simulink model "foc"  (R2021b)
settings: Solver=FixedStepAuto  StartTime=0.0  StopTime=20  FixedStep=Ts  MaxStep=1e-4  RelTol=1e-3  EnableMultiTasking=on
model workspace (MAT data in the model file):
  flux = 0.154
values from neighbouring files (symbols this model uses):
  currt_width = 200.0    [motor_parameters.sldd]
  Flux = 0.00103001    [motor_parameters.sldd]
  Ibus = 5.0    [motor_parameters.sldd]
  Ld = 2.235E-5    [motor_parameters.sldd]
  Lq = 2.567E-5    [motor_parameters.sldd]
  Ls = 2.235E-5    [motor_parameters.sldd]
  OPL_time = 3.0    [motor_parameters.sldd]
  Pn = 7.0    [motor_parameters.sldd]
  R = 0.083    [motor_parameters.sldd]
  Rs = 0.112    [motor_parameters.sldd]
  smo_l = 0.1    [motor_parameters.sldd]
  smo_m = 0.001    [motor_parameters.sldd]
  Ts = 0.0001    [motor_parameters.sldd]
  Ubus = 12.0    [motor_parameters.sldd]
undefined symbols (not defined in the file or in its folder): DiscIntNeverNeededParam, sigbuilder_block, spd_ki, spd_kp
libraries: slpidlib x6, simulink x3, mcbcontrolslib x3, mcbplantlib x1, autolibpmsmexterior x1
(part 2 of 2)

== system foc/FOC_Model/currloop/HFI_Observer/waichafa ==
  i_alpha_n : Inport
  i_beta_n : Inport  Port=2
  "   " : Product
  "    " : Product
  Discrete PID Controller : slpidlib/PID Controller  Controller=PI  Form=Parallel  TimeDomain=Discrete-time  UseExternalTs=off  SampleTime=-1  IntegratorMethod=Forward Euler  FilterMethod=Forward Euler  ControllerParametersSource=internal  P=100  I=15000  D=0  UseFilter=on  N=100  TunerSelectOption=Transfer Function Based (PID Tuner App)  InitialConditionSource=internal  InitialConditionForIntegrator=0  InitialConditionForFilter=0  DifferentiatorICPrevScaledInput=0  ExternalReset=none  TrackingMode=off  Kt=1  LimitOutput=off  SatLimitsSource=internal  UpperSaturationLimit=inf  LowerSaturationLimit=-inf  LinearizeAsGain=off  AntiWindupMode=none  Kb=1  POutMin=[]  POutMax=[]  IOutMin=[]  IOutMax=[]  DOutMin=[]  DOutMax=[]  NOutMin=[]  NOutMax=[]  SumOutMin=[]  SumOutMax=[]  SaturationOutMin=[]  SaturationOutMax=[]  PParamMin=[]  PParamMax=[]  IParamMin=[]  IParamMax=[]  DParamMin=[]  DParamMax=[]  NParamMin=[]  NParamMax=[]  KbParamMin=[]  KbParamMax=[]  KtParamMin=[]  KtParamMax=[]  KbOutMin=[]  KbOutMax=[]  KtOutMin=[]  KtOutMax=[]  IntegratorOutMin=[]  IntegratorOutMax=[]  FilterOutMin=[]  FilterOutMax=[]  SumI1OutMin=[]  SumI1OutMax=[]  SumI2OutMin=[]  SumI2OutMax=[]  SumI3OutMin=[]  SumI3OutMax=[]  SumI4OutMin=[]  SumI4OutMax=[]  SumDOutMin=[]  SumDOutMax=[]  DifferentiatorOutMin=[]  DifferentiatorOutMax=[]  FilterDiffOutCoefMin=[]  FilterDiffOutCoefMax=[]  ReciprocalOutMin=[]  ReciprocalOutMax=[]  SumDenOutMin=[]  SumDenOutMax=[]  SumNumOutMin=[]  SumNumOutMax=[]  DivideOutMin=[]  DivideOutMax=[]  UdiffTsProdOutMin=[]  UdiffTsProdOutMax=[]  NTsProdOutMin=[]  NTsProdOutMax=[]  UintegralTsProdOutMin=[]  UintegralTsProdOutMax=[]  UngainTsProdOutMin=[]  UngainTsProdOutMax=[]  IntegratorContinuousStateAttributes=''  IntegratorStateMustResolveToSignalObject=off  IntegratorRTWStateStorageClass=Auto  FilterContinuousStateAttributes=''  FilterStateMustResolveToSignalObject=off  FilterRTWStateStorageClass=Auto  ParallelPVariant=InternalParameters  IdealPVariant=Disabled  IVariant=InternalParameters  DVariant=Disabled  IntegratorVariant=Discrete  SatVariant=Disabled  AWVariant=Passthrough  PCopyVariant=Disabled  TRVariant=Disabled  FdbkBlocksVariant=Forward  IdealPFdbkVariant=Disabled  SatFdbkVariant=Disabled  DerivativeFilterVariant=Disabled  NVariant=Disabled  NCopyVariant=Disabled_SignalSpec  FilterICVariant=Disabled  IntegratorICVariant=InternalICs  ExternalResetVariant=Disabled  TRSumVariant=Passthrough  SumFdbkVariant=Disabled  SumVariant=Sum_PI  TsampFilterVariant=InternalTs  TsampNgainVariant=Passthrough  TsampIntegralVariant=Passthrough  ExternalSaturationOutDataTypeStr=Inherit: Same as second input
  Discrete-Time Integrator : DiscreteIntegrator  SampleTime=-1  ICPrevOutput=DiscIntNeverNeededParam  ICPrevScaledInput=DiscIntNeverNeededParam
  Fcn : Fcn  Expr=sin(u(1))
  Fcn1 : Fcn  Expr=cos(u(1))
  Fcn2 : Fcn  Expr=u(1)/sqrt(u(1)*u(1)+u(2)*u(2))
  Fcn3 : Fcn  Expr=u(2)/sqrt(u(1)*u(1)+u(2)*u(2))
  Mux : Mux  Inputs=2
  Scope : Scope  NumInputPorts=2
  Scope1 : Scope
  Sum9 : Sum  Inputs=-+
  theta : Outport  VectorParamsAs1DForOutWhenUnconnected=off
  we : Outport  Port=2  VectorParamsAs1DForOutWhenUnconnected=off
  wires:
  "   "/1 -> Sum9/2
  Fcn1/1 -> "   "/1
  "    "/1 -> Sum9/1
  Fcn/1 -> "    "/2
  i_alpha_n/1 -> Mux/1
  Mux/1 -> Fcn3/1, Fcn2/1
  Fcn2/1 -> Scope/1, "    "/1
  Discrete-Time Integrator/1 -> theta/1, Fcn/1, Fcn1/1
  Fcn3/1 -> "   "/2, Scope/2
  Sum9/1 -> Scope1/1, Discrete PID Controller/1
  Discrete PID Controller/1 -> we/1, Discrete-Time Integrator/1
  i_beta_n/1 -> Mux/2

== system foc/FOC_Model/currloop/If Action Subsystem2/If Action Subsystem ==
  Action Port : ActionPort  ActionPortLabel=if(u1 >= 0)
  Constant : Constant  Value=0  OutDataTypeStr=single
  Out1 : Outport
  wires:
  Constant/1 -> Out1/1

== system foc/FOC_Model/currloop/If Action Subsystem2/If Action Subsystem1 ==
  Action Port : ActionPort  ActionPortLabel=else
  Constant : Constant  Value=pi  OutDataTypeStr=single
  Out1 : Outport
  wires:
  Constant/1 -> Out1/1

== system foc/FOC_Model/currloop/SMO/PLL ==
  e_alpha_est : Inport
  e_beta_est : Inport  Port=2
  Constant : Constant  Value=2*pi  SampleTime=-1
  Cos : Trigonometry  Operator=cos
  Discrete-Time Integrator : DiscreteIntegrator  SampleTime=-1  ICPrevOutput=DiscIntNeverNeededParam  ICPrevScaledInput=DiscIntNeverNeededParam
  IIR Filter : mcbcontrolslib/IIR Filter  VariantControl=Low Pass Filter  VariantSelect=Low-pass  Filter_constant=0.0004  advancedSettings=on  Ts=1e-6  cutOff_freq=63.6875
      settings: SourceProductBaseCode=MT
  IIR Filter1 : mcbcontrolslib/IIR Filter  VariantControl=Low Pass Filter  VariantSelect=Low-pass  Filter_constant=0.0004  advancedSettings=on  Ts=1e-5  cutOff_freq=6.3687
      settings: SourceProductBaseCode=MT
  Mod : Math  Operator=mod  SaturateOnIntegerOverflow=on
  PLL : Subsystem
      mask Display: disp('PI')
  Product : Product
  Product1 : Product
  Scope : Scope
  Sin : Trigonometry
  Sum : Sum  Inputs=--
  theta_est : Outport
  we_est : Outport  Port=2
  wires:
  e_alpha_est/1 -> Product/2
  Cos/1 -> Product/1
  Product/1 -> Sum/1
  e_beta_est/1 -> Product1/1
  Product1/1 -> Sum/2
  Sin/1 -> Product1/2
  Discrete-Time Integrator/1 -> Mod/1, Cos/1, Sin/1
  Sum/1 -> PLL/1(e)
  PLL/1(output) -> IIR Filter1/1, Discrete-Time Integrator/1
  IIR Filter1/1 -> Scope/1, we_est/1
  Mod/1 -> theta_est/1
  Constant/1 -> Mod/2

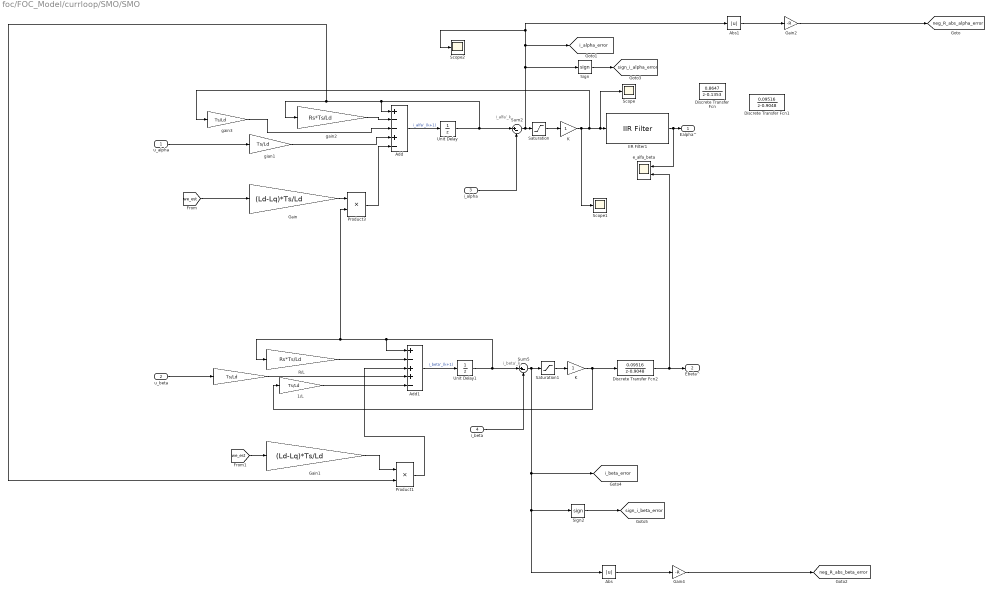
== system foc/FOC_Model/currloop/SMO/SMO ==
  note: i_alfa'_k
  note: i_beta'_k
  u_alpha : Inport  OutDataTypeStr=single
  u_beta : Inport  Port=2  OutDataTypeStr=single
  i_alpha : Inport  Port=3  OutDataTypeStr=single
  i_beta : Inport  Port=4  OutDataTypeStr=single
  " " : Gain  Gain=Ts/Ld
  " 1/L " : Gain  Gain=Ts/Ld
  Abs : Abs
  Abs1 : Abs
  Add : Sum  Inputs=+--+-  OutDataTypeStr=single
  Add1 : Sum  Inputs=+-++-
  Discrete Transfer Fcn : DiscreteTransferFcn  Numerator=[0.8647]  Denominator=[1 -0.1353]
  Discrete Transfer Fcn1 : DiscreteTransferFcn  Numerator=[0.09516]  Denominator=[1 -0.9048]
  Discrete Transfer Fcn2 : DiscreteTransferFcn  Numerator=[0.09516]  Denominator=[1 -0.9048]
  Gain : Gain  Gain=(Ld-Lq)*Ts/Ld
  Gain1 : Gain  Gain=(Ld-Lq)*Ts/Ld
  Gain2 : Gain  Gain=-R
  Gain4 : Gain  Gain=-R
  IIR Filter1 : mcbcontrolslib/IIR Filter  VariantControl=Low Pass Filter  VariantSelect=Low-pass  Filter_constant=0.1  advancedSettings=on  Ts=1e-4  cutOff_freq=176.8388
      settings: SourceProductBaseCode=MT
  K : Gain
  "K " : Gain
  Product1 : Product  RndMeth=Zero
  Product3 : Product  RndMeth=Zero
  "R/L " : Gain  Gain=Rs*Ts/Ld
  Saturation : Saturate  UpperLimit=2  LowerLimit=-2
  Saturation1 : Saturate  UpperLimit=2  LowerLimit=-2
  Scope : Scope
  Scope1 : Scope
  Scope2 : Scope
  Sign : Signum  ZeroCross=off
  Sign2 : Signum  ZeroCross=off
  Sum2 : Sum  Inputs=|+-
  Sum5 : Sum  Inputs=|+-
  Unit Delay : UnitDelay  SampleTime=-1  HasFrameUpgradeWarning=on
  Unit Delay1 : UnitDelay  SampleTime=-1  HasFrameUpgradeWarning=on
  e_alfa_beta : Scope  NumInputPorts=2
  gain2 : Gain  Gain=Rs*Ts/Ld  OutDataTypeStr=single
  gain3 : Gain  Gain=Ts/Ld
  gian1 : Gain  Gain=Ts/Ld
  Ealpha^ : Outport
  Ebeta^ : Outport  Port=2
  tag scope: i_alpha_error=global, i_beta_error=global, neg_R_abs_alpha_error=global, neg_R_abs_beta_error=global, sign_i_alpha_error=global, sign_i_beta_error=global
  wires:
  Saturation/1 -> K/1
  K/1 -> Scope1/1, IIR Filter1/1, Scope/1, gain3/1
  Unit Delay1/1 -> Add1/1, Product3/2, "R/L "/1, Sum5/1
  Saturation1/1 -> "K "/1
  " "/1 -> Add1/4
  "R/L "/1 -> Add1/2
  [we_est] -> Gain/1
  Gain/1 -> Product3/1
  Gain1/1 -> Product1/1
  [we_est] -> Gain1/1
  Product1/1 -> Add1/3
  Unit Delay/1 -> Product1/2, gain2/1, Add/1, Sum2/1
  Add/1 -> Unit Delay/1  "i_alfa'_(k+1)"
  gain2/1 -> Add/2
  gian1/1 -> Add/4
  Product3/1 -> Add/5
  gain3/1 -> Add/3
  Add1/1 -> Unit Delay1/1  "i_beta'_(k+1)"
  " 1/L "/1 -> Add1/5
  Sum2/1 -> Sign/1, [i_alpha_error], Scope2/1, Abs1/1, Saturation/1
  Gain2/1 -> [neg_R_abs_alpha_error]
  Abs1/1 -> Gain2/1
  Abs/1 -> Gain4/1
  Gain4/1 -> [neg_R_abs_beta_error]
  Sum5/1 -> Sign2/1, Abs/1, [i_beta_error], Saturation1/1
  Sign/1 -> [sign_i_alpha_error]
  Sign2/1 -> [sign_i_beta_error]
  u_alpha/1 -> gian1/1
  u_beta/1 -> " "/1
  i_alpha/1 -> Sum2/2
  i_beta/1 -> Sum5/2
  "K "/1 -> Discrete Transfer Fcn2/1, " 1/L "/1
  Discrete Transfer Fcn2/1 -> e_alfa_beta/2, Ebeta^/1
  IIR Filter1/1 -> e_alfa_beta/1, Ealpha^/1

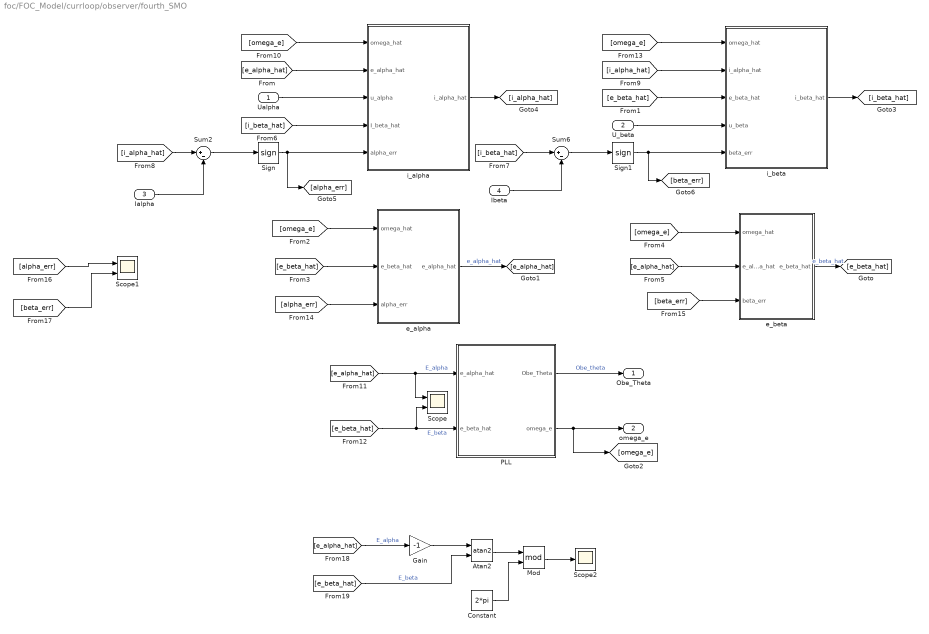
== system foc/FOC_Model/currloop/observer/fourth_SMO ==
  Ualpha : Inport
  U_beta : Inport  Port=2
  Ialpha : Inport  Port=3
  Ibeta : Inport  Port=4
  Atan2 : Trigonometry  Operator=atan2
  Constant : Constant  Value=2*pi  OutDataTypeStr=single
  Gain : Gain  Gain=-1  OutDataTypeStr=single
  Mod : Math  Operator=mod  SaturateOnIntegerOverflow=on
  PLL : Subsystem
  Scope : Scope  NumInputPorts=2
  Scope1 : Scope  NumInputPorts=2
  Scope2 : Scope
  Sign : Signum
  Sign1 : Signum
  Sum2 : Sum  Inputs=|+-
  Sum6 : Sum  Inputs=|+-
  e_alpha : Subsystem
  e_beta : Subsystem
  i_alpha : Subsystem
  i_beta : Subsystem
  Obe_Theta : Outport
  omega_e : Outport  Port=2
  wires:
  Sum6/1 -> Sign1/1
  Sum2/1 -> Sign/1
  Sign/1 -> i_alpha/5(alpha_err), [alpha_err]
  Ialpha/1 -> Sum2/2
  Sign1/1 -> [beta_err], i_beta/5(beta_err)
  Ibeta/1 -> Sum6/2
  i_alpha/1(i_alpha_hat) -> [i_alpha_hat]
  [e_alpha_hat] -> i_alpha/2(e_alpha_hat)
  Ualpha/1 -> i_alpha/3(u_alpha)
  [e_beta_hat] -> i_beta/3(e_beta_hat)
  U_beta/1 -> i_beta/4(u_beta)
  i_beta/1(i_beta_hat) -> [i_beta_hat]
  [i_beta_hat] -> i_alpha/4(I_beta_hat)
  [i_beta_hat] -> Sum6/1
  [i_alpha_hat] -> Sum2/1
  [i_alpha_hat] -> i_beta/2(i_alpha_hat)
  [omega_e] -> e_alpha/1(omega_hat)
  [e_beta_hat] -> e_alpha/2(e_beta_hat)
  [omega_e] -> e_beta/1(omega_hat)
  [e_alpha_hat] -> e_beta/2(e_alpha_hat)
  [omega_e] -> i_alpha/1(omega_hat)
  e_beta/1(e_beta_hat) -> [e_beta_hat]  "e_beta_hat"
  e_alpha/1(e_alpha_hat) -> [e_alpha_hat]  "e_alpha_hat"
  [e_alpha_hat] -> Scope/1, PLL/1(e_alpha_hat)  "E_alpha"
  [e_beta_hat] -> Scope/2, PLL/2(e_beta_hat)  "E_beta"
  PLL/2(omega_e) -> [omega_e], omega_e/1
  [omega_e] -> i_beta/1(omega_hat)
  PLL/1(Obe_Theta) -> Obe_Theta/1  "Obe_theta"
  [alpha_err] -> e_alpha/3(alpha_err)
  [beta_err] -> e_beta/3(beta_err)
  [alpha_err] -> Scope1/1
  [beta_err] -> Scope1/2
  [e_alpha_hat] -> Gain/1  "E_alpha"
  Gain/1 -> Atan2/1
  [e_beta_hat] -> Atan2/2  "E_beta"
  Atan2/1 -> Mod/1
  Constant/1 -> Mod/2
  Mod/1 -> Scope2/1

== system foc/FOC_Model/currloop/svpwm/Anti_Park_Trans ==
  note: Valpha = ud*cos(theta) - uq*sin(theta);
      | Vbeta = ud*sin(theta) + uq*cos(theta);
  ud : Inport  OutDataTypeStr=single
  uq : Inport  Port=2  OutDataTypeStr=single
  theta : Inport  Port=3
  Add : Sum  Inputs=+-
  Add1 : Sum
  Cos : Trigonometry  Operator=cos
  Product{,1..3} (4 alike) : Product
  Scope : Scope  NumInputPorts=2
  Sin : Trigonometry
  ualpha : Outport  OutDataTypeStr=single
  ubeta : Outport  Port=2  OutDataTypeStr=single
  wires:
  Add/1 -> ualpha/1
  ud/1 -> Product2/1, Product/1
  Cos/1 -> Product/2, Scope/2, Product3/2
  Product/1 -> Add/1
  uq/1 -> Product3/1, Product1/1
  theta/1 -> Sin/1, Cos/1
  Product1/1 -> Add/2
  Product2/1 -> Add1/1
  Product3/1 -> Add1/2
  Add1/1 -> ubeta/1
  Sin/1 -> Scope/1, Product2/2, Product1/2

== system foc/FOC_Model/currloop/SMO/PLL/PLL ==
  e : Inport
  Add : Sum
  Discrete-Time Integrator : DiscreteIntegrator  SampleTime=-1  ICPrevOutput=DiscIntNeverNeededParam  ICPrevScaledInput=DiscIntNeverNeededParam
  Ki : Gain  Gain=36000
  Kp : Gain  Gain=540
  Saturation : Saturate  UpperLimit=2000  LowerLimit=-2000
  output : Outport
  wires:
  Ki/1 -> Discrete-Time Integrator/1
  e/1 -> Kp/1, Ki/1
  Saturation/1 -> output/1
  Discrete-Time Integrator/1 -> Add/2
  Kp/1 -> Add/1
  Add/1 -> Saturation/1

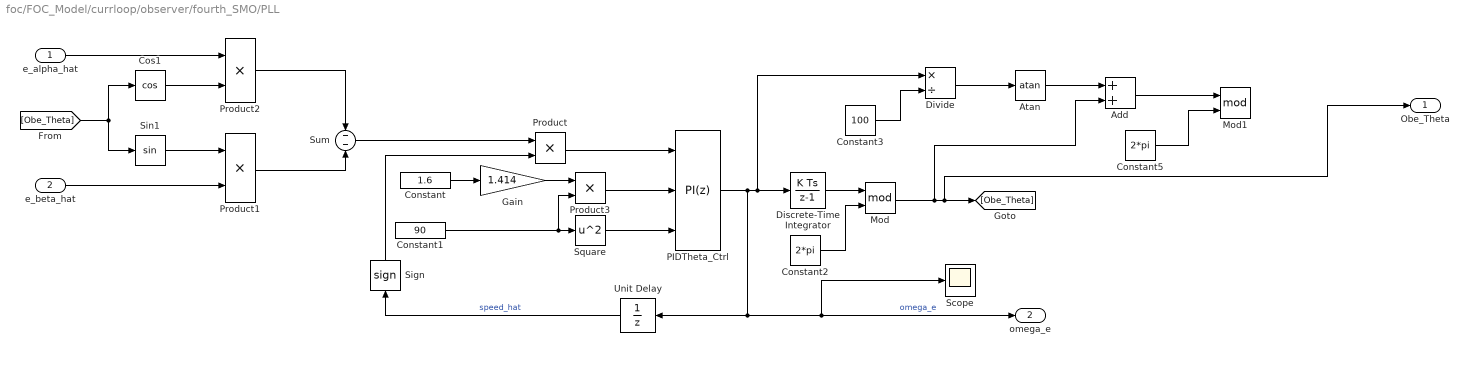
== system foc/FOC_Model/currloop/observer/fourth_SMO/PLL ==
  e_alpha_hat : Inport
  e_beta_hat : Inport  Port=2
  Add : Sum
  Atan : Trigonometry  Operator=atan
  Constant : Constant  Value=1.6  OutDataTypeStr=single  SampleTime=-1
  Constant1 : Constant  Value=90  OutDataTypeStr=single  SampleTime=-1
  Constant2 : Constant  Value=2*pi  OutDataTypeStr=single  SampleTime=Ts
  Constant3 : Constant  Value=100
  Constant5 : Constant  Value=2*pi  OutDataTypeStr=single  SampleTime=Ts
  Cos1 : Trigonometry  Operator=cos
  Discrete-Time Integrator : DiscreteIntegrator  SampleTime=Ts  ICPrevOutput=DiscIntNeverNeededParam  ICPrevScaledInput=DiscIntNeverNeededParam
  Divide : Product  Inputs=*/  OutDataTypeStr=single
  Gain : Gain  Gain=1.414
  Mod : Math  Operator=mod  SignedPower=on  SaturateOnIntegerOverflow=on
  Mod1 : Math  Operator=mod  SaturateOnIntegerOverflow=on
  PIDTheta_Ctrl : slpidlib/PID Controller  Controller=PI  Form=Parallel  TimeDomain=Discrete-time  UseExternalTs=off  SampleTime=-1  IntegratorMethod=Forward Euler  FilterMethod=Forward Euler  ControllerParametersSource=external  P=2*0.707*100  I=100*100  D=0  UseFilter=on  N=100  TunerSelectOption=Transfer Function Based (PID Tuner App)  ZeroCross=off  InitialConditionSource=internal  InitialConditionForIntegrator=50  InitialConditionForFilter=0  DifferentiatorICPrevScaledInput=0  ExternalReset=none  TrackingMode=off  Kt=1  LimitOutput=on  SatLimitsSource=internal  UpperSaturationLimit=3000  LowerSaturationLimit=-3000  LinearizeAsGain=off  AntiWindupMode=clamping  Kb=50  POutMin=[]  POutMax=[]  IOutMin=[]  IOutMax=[]  DOutMin=[]  DOutMax=[]  NOutMin=[]  NOutMax=[]  SumOutMin=[]  SumOutMax=[]  SaturationOutDataTypeStr=Inherit: Inherit via back propagation  SaturationOutMin=[]  SaturationOutMax=[]  PParamMin=[]  PParamMax=[]  IParamMin=[]  IParamMax=[]  DParamMin=[]  DParamMax=[]  NParamMin=[]  NParamMax=[]  KbParamMin=[]  KbParamMax=[]  KtParamMin=[]  KtParamMax=[]  KbOutMin=[]  KbOutMax=[]  KtOutMin=[]  KtOutMax=[]  IntegratorOutMin=[]  IntegratorOutMax=[]  FilterOutMin=[]  FilterOutMax=[]  SumI1OutMin=[]  SumI1OutMax=[]  SumI2OutMin=[]  SumI2OutMax=[]  SumI3OutMin=[]  SumI3OutMax=[]  SumI4OutMin=[]  SumI4OutMax=[]  SumDOutMin=[]  SumDOutMax=[]  DifferentiatorOutMin=[]  DifferentiatorOutMax=[]  FilterDiffOutCoefMin=[]  FilterDiffOutCoefMax=[]  ReciprocalOutMin=[]  ReciprocalOutMax=[]  SumDenOutMin=[]  SumDenOutMax=[]  SumNumOutMin=[]  SumNumOutMax=[]  DivideOutMin=[]  DivideOutMax=[]  UdiffTsProdOutMin=[]  UdiffTsProdOutMax=[]  NTsProdOutMin=[]  NTsProdOutMax=[]  UintegralTsProdOutMin=[]  UintegralTsProdOutMax=[]  UngainTsProdOutMin=[]  UngainTsProdOutMax=[]  IntegratorContinuousStateAttributes=''  IntegratorStateMustResolveToSignalObject=off  IntegratorRTWStateStorageClass=Auto  FilterContinuousStateAttributes=''  FilterStateMustResolveToSignalObject=off  FilterRTWStateStorageClass=Auto  ParallelPVariant=ExternalParameters  IdealPVariant=Disabled  IVariant=ExternalParameters  DVariant=Disabled  IntegratorVariant=Discrete  SatVariant=Enabled  AWVariant=DiscClampingParallel  PCopyVariant=Disabled  TRVariant=Disabled  FdbkBlocksVariant=Forward  IdealPFdbkVariant=Disabled  SatFdbkVariant=Disabled  DerivativeFilterVariant=Disabled  NVariant=Disabled  NCopyVariant=Disabled_SignalSpec  FilterICVariant=Disabled  IntegratorICVariant=InternalICs  ExternalResetVariant=Disabled  TRSumVariant=Passthrough  SumFdbkVariant=Disabled  SumVariant=Sum_PI  TsampFilterVariant=InternalTs  TsampNgainVariant=Passthrough  TsampIntegralVariant=Passthrough  ExternalSaturationOutDataTypeStr=Inherit: Same as second input
  Product{,1..3} (4 alike) : Product
  Scope : Scope
  Sign : Signum
  Sin1 : Trigonometry
  Square : Math  Operator=square  SignedPower=on  SaturateOnIntegerOverflow=on
  Sum : Sum  Inputs=-|-
  Unit Delay : UnitDelay  SampleTime=-1  HasFrameUpgradeWarning=on
  Obe_Theta : Outport
  omega_e : Outport  Port=2
  wires:
  Product/1 -> PIDTheta_Ctrl/1
  Sum/1 -> Product/1
  Product1/1 -> Sum/2
  Product2/1 -> Sum/1
  Unit Delay/1 -> Sign/1  "speed_hat"
  Sign/1 -> Product/2
  PIDTheta_Ctrl/1 -> Divide/1, Discrete-Time Integrator/1, Scope/1, omega_e/1, Unit Delay/1  "omega_e"
  Constant/1 -> Gain/1
  Constant1/1 -> Product3/2, Square/1
  Square/1 -> PIDTheta_Ctrl/3
  Gain/1 -> Product3/1
  Product3/1 -> PIDTheta_Ctrl/2
  Mod/1 -> Obe_Theta/1, [Obe_Theta], Add/2
  Discrete-Time Integrator/1 -> Mod/1
  Constant2/1 -> Mod/2
  e_alpha_hat/1 -> Product2/1
  Cos1/1 -> Product2/2
  Sin1/1 -> Product1/1
  e_beta_hat/1 -> Product1/2
  Constant3/1 -> Divide/2
  Divide/1 -> Atan/1
  Atan/1 -> Add/1
  Add/1 -> Mod1/1
  Constant5/1 -> Mod1/2
  [Obe_Theta] -> Cos1/1, Sin1/1

== system foc/FOC_Model/currloop/observer/fourth_SMO/e_alpha ==
  omega_hat : Inport
  e_beta_hat : Inport  Port=2
  alpha_err : Inport  Port=3
  Add2 : Sum  Inputs=-+
  Constant : Constant  Value=Ld  OutDataTypeStr=single
  Discrete-Time Integrator : DiscreteIntegrator  SampleTime=Ts  ICPrevOutput=DiscIntNeverNeededParam  ICPrevScaledInput=DiscIntNeverNeededParam
  Divide : Product  Inputs=*/
  Gain3 : Gain  Gain=smo_m
  Product2 : Product
  Unit Delay2 : UnitDelay  SampleTime=-1  HasFrameUpgradeWarning=on
  e_alpha_hat : Outport
  wires:
  Unit Delay2/1 -> e_alpha_hat/1
  omega_hat/1 -> Product2/1
  Product2/1 -> Add2/1
  Discrete-Time Integrator/1 -> Unit Delay2/1
  e_beta_hat/1 -> Product2/2
  Divide/1 -> Add2/2
  alpha_err/1 -> Gain3/1
  Constant/1 -> Divide/2
  Gain3/1 -> Divide/1
  Add2/1 -> Discrete-Time Integrator/1

== system foc/FOC_Model/currloop/observer/fourth_SMO/e_beta ==
  omega_hat : Inport
  e_alpha_hat : Inport  Port=2
  beta_err : Inport  Port=3
  Add3 : Sum
  Constant : Constant  Value=Ld  OutDataTypeStr=single
  Discrete-Time Integrator : DiscreteIntegrator  SampleTime=Ts  ICPrevOutput=DiscIntNeverNeededParam  ICPrevScaledInput=DiscIntNeverNeededParam
  Divide : Product  Inputs=*/
  Gain1 : Gain  Gain=smo_m
  Product3 : Product
  Unit Delay3 : UnitDelay  SampleTime=-1  HasFrameUpgradeWarning=on
  e_beta_hat : Outport
  wires:
  Discrete-Time Integrator/1 -> Unit Delay3/1
  Product3/1 -> Add3/1
  Unit Delay3/1 -> e_beta_hat/1
  omega_hat/1 -> Product3/1
  e_alpha_hat/1 -> Product3/2
  Constant/1 -> Divide/2
  beta_err/1 -> Gain1/1
  Divide/1 -> Add3/2
  Gain1/1 -> Divide/1
  Add3/1 -> Discrete-Time Integrator/1

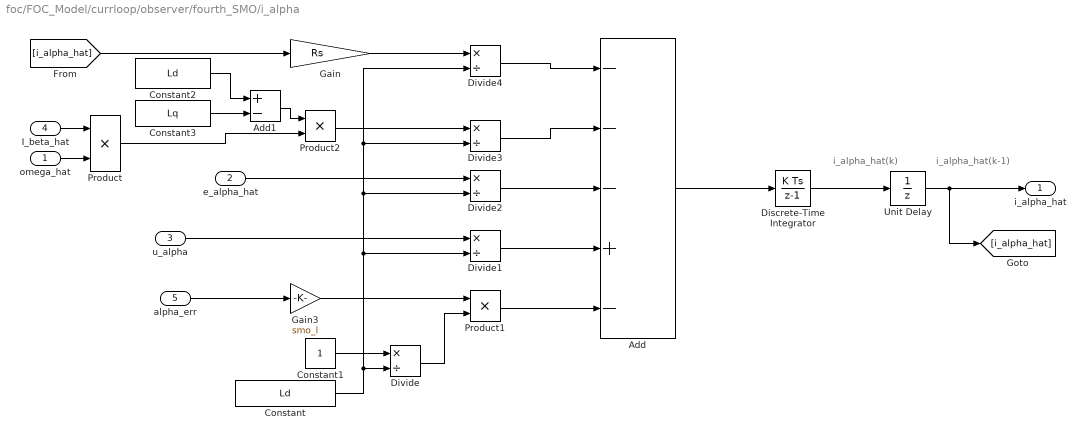
== system foc/FOC_Model/currloop/observer/fourth_SMO/i_alpha ==
  note: i_alpha_hat(k)
  note: i_alpha_hat(k-1)
  omega_hat : Inport
  e_alpha_hat : Inport  Port=2
  u_alpha : Inport  Port=3
  I_beta_hat : Inport  Port=4
  alpha_err : Inport  Port=5
  Add : Sum  Inputs=---+-
  Add1 : Sum  Inputs=+-
  Constant : Constant  Value=Ld  OutDataTypeStr=single
  Constant1 : Constant  OutDataTypeStr=single
  Constant2 : Constant  Value=Ld  OutDataTypeStr=single
  Constant3 : Constant  Value=Lq  OutDataTypeStr=single
  Discrete-Time Integrator : DiscreteIntegrator  SampleTime=Ts  ICPrevOutput=DiscIntNeverNeededParam  ICPrevScaledInput=DiscIntNeverNeededParam
  Divide{,1..4} (5 alike) : Product  Inputs=*/
  Gain : Gain  Gain=Rs
  Gain3 : Gain  Gain=smo_l
  Product : Product
  Product1 : Product
  Product2 : Product
  Unit Delay : UnitDelay  SampleTime=-1  HasFrameUpgradeWarning=on
  i_alpha_hat : Outport
  wires:
  Divide3/1 -> Add/2
  Product1/1 -> Add/5
  Add/1 -> Discrete-Time Integrator/1
  I_beta_hat/1 -> Product/1
  Unit Delay/1 -> [i_alpha_hat], i_alpha_hat/1
  u_alpha/1 -> Divide1/1
  Divide1/1 -> Add/4
  Discrete-Time Integrator/1 -> Unit Delay/1
  omega_hat/1 -> Product/2
  Divide2/1 -> Add/3
  e_alpha_hat/1 -> Divide2/1
  alpha_err/1 -> Gain3/1
  [i_alpha_hat] -> Gain/1
  Gain3/1 -> Product1/1
  Constant/1 -> Divide2/2, Divide3/2, Divide4/2, Divide1/2, Divide/2
  Divide/1 -> Product1/2
  Constant1/1 -> Divide/1
  Constant2/1 -> Add1/1
  Constant3/1 -> Add1/2
  Product/1 -> Product2/2
  Add1/1 -> Product2/1
  Product2/1 -> Divide3/1
  Divide4/1 -> Add/1
  Gain/1 -> Divide4/1

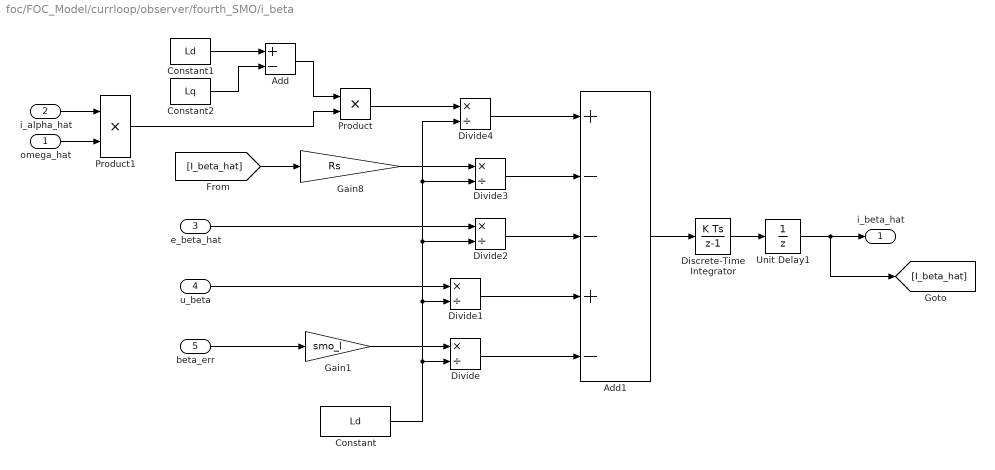
== system foc/FOC_Model/currloop/observer/fourth_SMO/i_beta ==
  omega_hat : Inport
  i_alpha_hat : Inport  Port=2
  e_beta_hat : Inport  Port=3
  u_beta : Inport  Port=4
  beta_err : Inport  Port=5
  Add : Sum  Inputs=+-
  Add1 : Sum  Inputs=+--+-
  Constant : Constant  Value=Ld  OutDataTypeStr=single
  Constant1 : Constant  Value=Ld  OutDataTypeStr=single
  Constant2 : Constant  Value=Lq  OutDataTypeStr=single
  Discrete-Time Integrator : DiscreteIntegrator  SampleTime=Ts  ICPrevOutput=DiscIntNeverNeededParam  ICPrevScaledInput=DiscIntNeverNeededParam
  Divide{,1..4} (5 alike) : Product  Inputs=*/
  Gain1 : Gain  Gain=smo_l
  Gain8 : Gain  Gain=Rs
  Product : Product
  Product1 : Product
  Unit Delay1 : UnitDelay  SampleTime=-1  HasFrameUpgradeWarning=on
  i_beta_hat : Outport
  wires:
  u_beta/1 -> Divide1/1
  Add1/1 -> Discrete-Time Integrator/1
  i_alpha_hat/1 -> Product1/1
  Discrete-Time Integrator/1 -> Unit Delay1/1
  e_beta_hat/1 -> Divide2/1
  Unit Delay1/1 -> i_beta_hat/1, [I_beta_hat]
  omega_hat/1 -> Product1/2
  [I_beta_hat] -> Gain8/1
  Gain1/1 -> Divide/1
  beta_err/1 -> Gain1/1
  Divide/1 -> Add1/5
  Constant/1 -> Divide4/2, Divide3/2, Divide2/2, Divide1/2, Divide/2
  Divide1/1 -> Add1/4
  Divide2/1 -> Add1/3
  Divide3/1 -> Add1/2
  Gain8/1 -> Divide3/1
  Constant1/1 -> Add/1
  Constant2/1 -> Add/2
  Divide4/1 -> Add1/1
  Product/1 -> Divide4/1
  Product1/1 -> Product/2
  Add/1 -> Product/1

== matlab function foc/FOC_Model/currloop/svpwm/foc ==
  data: Valpha input; Tcmp1 output; Vbeta input; Udc input; Tpwm input; Tcmp2 output; Tcmp3 output; sector output
function [Tcmp1,Tcmp2,Tcmp3,sector] = fcn(Valpha,Vbeta,Udc,Tpwm)
%#codegen

sector = single(0);
Tcmp1 = single(0);
Tcmp2 = single(0);
Tcmp3 = single(0);

%========Parameters statement================

    Vref1 = Vbeta;							                   
    Vref2 = (sqrt(3)*Valpha - Vbeta)/2; 				    
    Vref3 = (-sqrt(3)*Valpha - Vbeta)/2;					
   
 %========Sector calculation=================

  if (Vref1>0)
	   sector = single(1);
  end
  if (Vref2>0)
	   sector = sector+single(2);
  end
  if (Vref3>0)
       sector = sector+single(4);
  end

%======== X Y Z calculation===================

X = sqrt(3)*Vbeta*Tpwm/Udc;
Y = Tpwm/Udc*(3/2*Valpha+sqrt(3)/2*Vbeta);
Z = Tpwm/Udc*(-3/2*Valpha+sqrt(3)/2*Vbeta);	         

%==========Duty ratio calculation================
switch (sector)   
    case 1
        T1 = Z; T2 = Y; 
	case 2
        T1 = Y; T2 = -X; 
	case 3
        T1 = -Z; T2 = X; 
	case 4
        T1 = -X; T2 = Z;
	case 5
        T1 = X; T2 = -Y;
    otherwise
        T1 = -Y; T2 = -Z;
end

if T1+T2 > Tpwm
    T1 = T1/(T1+T2);
    T2 = T2/(T1+T2);
else
    T1 = T1;
    T2 = T2;
end
ta = (Tpwm-(T1+T2))/4.0;
tb = ta+T1/2;
tc = tb+T2/2;

%==========Duty ratio calculation================
switch (sector)
    case 1 
        Tcmp1=tb;
        Tcmp2=ta;
        Tcmp3=tc; 
        
    case 2 
        Tcmp1=ta;
        Tcmp2=tc;
        Tcmp3=tb; 
       
    case 3 
        Tcmp1=ta;
        Tcmp2=tb;
        Tcmp3=tc; 
        
    case 4 
        Tcmp1=tc;
        Tcmp2=tb;
        Tcmp3=ta;
        
    case 5 
        Tcmp1=tc;
        Tcmp2=ta;
        Tcmp3=tb;
        
   case 6
       Tcmp1=tb;
       Tcmp2=tc;
       Tcmp3=ta;
end
end

== stateflow chart foc/FOC_Model/currloop/Chart ==
  state IDLE
    HFI_STATE=0;
    HFI_RUN=0;
  state HFI_START
    HFI_STATE=1;
    HFI_RUN=0;
  state INJECT_POSIT
    HFI_STATE=2;
    HFI_RUN=1;
  state INJECT_NEGAT
    HFI_STATE=3;
    HFI_RUN=1;
  state HFI_NS
    HFI_STATE=4;
    HFI_RUN=0;
  state HFI_OVER1
    HFI_STATE=5;
    HFI_RUN=0;
  (default) -> IDLE
  IDLE -> HFI_START : [HFI_SWITCH==1]
  HFI_START -> INJECT_POSIT [order 1] : [after(0.1,sec)]
  INJECT_POSIT -> INJECT_NEGAT [order 1] : [after(0.002,sec)]
  INJECT_NEGAT -> HFI_NS [order 1] : [after(0.002,sec)]
  HFI_NS -> HFI_OVER1 [order 2] : [after(0.01,sec)]
  HFI_START -> IDLE [order 2] : [HFI_SWITCH==0]
  INJECT_POSIT -> IDLE [order 2] : [HFI_SWITCH==0]
  INJECT_NEGAT -> IDLE [order 2] : [HFI_SWITCH==0]
  HFI_NS -> IDLE [order 1] : [HFI_SWITCH==0]
  HFI_OVER1 -> IDLE : [HFI_SWITCH==0]
  data: HFI_STATE output; HFI_SWITCH input; HFI_RUN output

== stateflow chart foc/FOC_Model/Motor_State/Chart1 ==
  state IDLE
    Motor_state = 1;
    soure = 0;
  state AlignStage
    Motor_state = 2;
    soure = 0;
  state OpenStage
    Motor_state = 3;
    soure = 0;
  state RunStage
    Motor_state = 4;
    soure = 1;
  (default) -> IDLE
  OpenStage -> RunStage [order 2] : [after(OPL_time,sec) ]
  IDLE -> AlignStage : [Motor_OnOff ==1]
  AlignStage -> OpenStage [order 1] : [after(0.1,sec)]
  RunStage -> IDLE : [Motor_OnOff ==0]
  OpenStage -> IDLE [order 1] : [Motor_OnOff ==0]
  AlignStage -> IDLE [order 2] : [Motor_OnOff == 0]
  data: Motor_OnOff input; Motor_state output; Spd_switch input; OPL_time input; soure output single
